simulink model "problem4p43"  (R2022a)
settings: Solver=VariableStepAuto  StartTime=0.0  StopTime=5  RelTol=1e-12
settings Model: Creator=ianmf  LastModifiedBy=ianmf

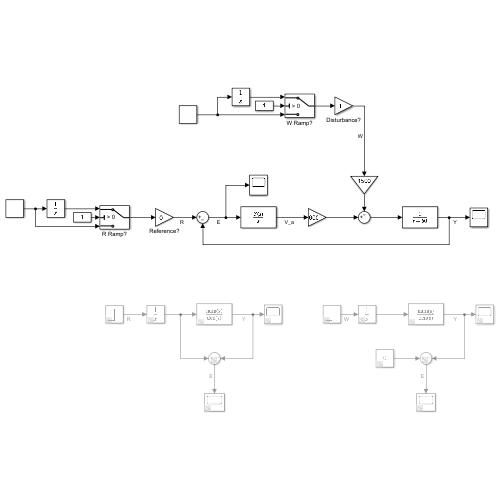
[thumbnail: Simulink's stored preview of the top-level diagram]
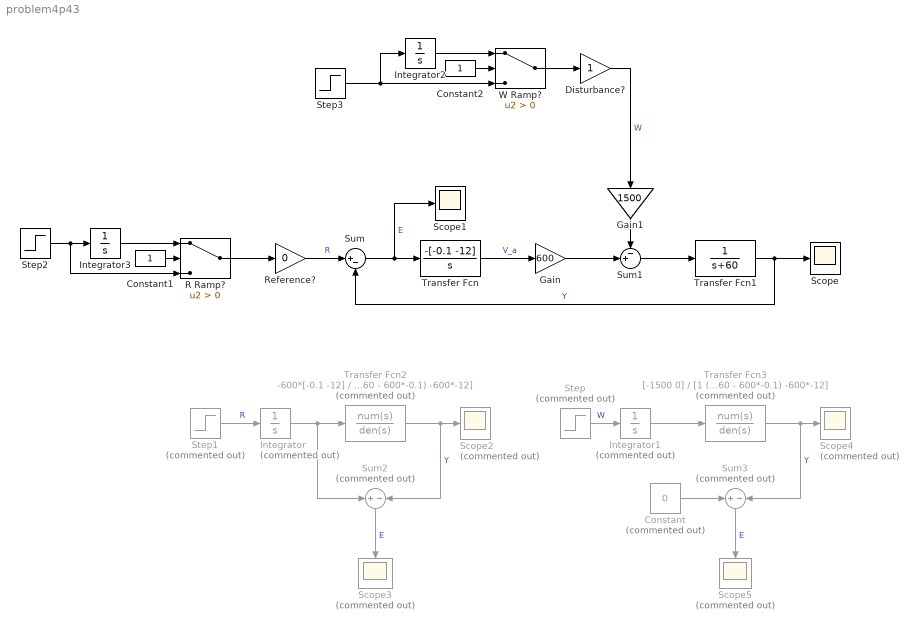
== system problem4p43 ==
  Constant : Constant  Commented=on  Value=0
  Constant1 : Constant
  Constant2 : Constant
  Disturbance? : Gain
  Gain : Gain  Gain=600
  Gain1 : Gain  Gain=1500
  Integrator : Integrator  Commented=on
  Integrator1 : Integrator  Commented=on
  Integrator2 : Integrator
  Integrator3 : Integrator
  R Ramp? : Switch  Criteria=u2 > Threshold  SaturateOnIntegerOverflow=off  InputSameDT=off
  Reference? : Gain  Gain=0
  Scope : Scope
  Scope1 : Scope
  Scope{2..5} (4 alike) : Scope  Commented=on
  Step : Step  Commented=on  Time=0  SampleTime=0
  Step1 : Step  Commented=on  Time=0  SampleTime=0
  Step2 : Step  Time=0  SampleTime=0
  Step3 : Step  Time=0  SampleTime=0
  Sum : Sum  Inputs=|+-
  Sum1 : Sum  Inputs=-+|
  Sum2 : Sum  Commented=on  Inputs=+|-
  Sum3 : Sum  Commented=on  Inputs=+|-
  Transfer Fcn : TransferFcn  Numerator=-[-0.1 -12]  Denominator=[1 0]
  Transfer Fcn1 : TransferFcn  Denominator=[1 60]
  Transfer Fcn2 : TransferFcn  Commented=on  Numerator=-600*[-0.1 -12]  Denominator=[1 (60 - 600*-0.1) -600*-12]
  Transfer Fcn3 : TransferFcn  Commented=on  Numerator=[-1500 0]  Denominator=[1 (60 - 600*-0.1) -600*-12]
  W Ramp? : Switch  Criteria=u2 > Threshold  SaturateOnIntegerOverflow=off  InputSameDT=off
  wires:
  Step2/1 -> R Ramp?/3, Integrator3/1
  Sum/1 -> Scope1/1, Transfer Fcn/1  "E"
  Transfer Fcn/1 -> Gain/1  "V_a"
  Gain/1 -> Sum1/2
  Integrator2/1 -> W Ramp?/1
  Gain1/1 -> Sum1/1
  Sum1/1 -> Transfer Fcn1/1
  Transfer Fcn1/1 -> Sum/2, Scope/1  "Y"
  Transfer Fcn2/1 -> Sum2/2, Scope2/1  "Y"
  Sum2/1 -> Scope3/1  "E"
  Sum3/1 -> Scope5/1  "E"
  Transfer Fcn3/1 -> Sum3/2, Scope4/1  "Y"
  Step/1 -> Integrator1/1  "W"
  Constant/1 -> Sum3/1
  Step1/1 -> Integrator/1  "R"
  Step3/1 -> W Ramp?/3, Integrator2/1
  Integrator/1 -> Sum2/1, Transfer Fcn2/1
  Integrator1/1 -> Transfer Fcn3/1
  Reference?/1 -> Sum/1  "R"
  W Ramp?/1 -> Disturbance?/1
  Integrator3/1 -> R Ramp?/1
  R Ramp?/1 -> Reference?/1
  Constant1/1 -> R Ramp?/2
  Constant2/1 -> W Ramp?/2
  Disturbance?/1 -> Gain1/1  "W"
